simulink library "animation_cl"  (R2018b)
settings: Solver=VariableStepAuto  StartTime=0.0  StopTime=10.0  RelTol=1e-3
values from neighbouring files (symbols this model uses):
  zenith = 90-elevation    [animation_init.m]
libraries: vrlib x3, eulAng2RotMat_ul x1, dspvision x1
settings Model: Creator=mcobb  LastModifiedBy=mcobb

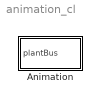
== system animation_cl ==
  Animation : Subsystem  mask{animSampleTime=0.1, elevation=75, radius=400, vidLogEnbl=on, vidDims=[240 480]}
      mask prompts: animSampleTime "Animation Sample Time"; vidLogEnbl "Enable"; vidDims "Video Dimensions"
      mask init:
      | animation_init
      mask DialogControl ParameterGroupVar Prompt: Viewpoint Specification
      mask DialogControl Container3 Prompt: Video File Logging

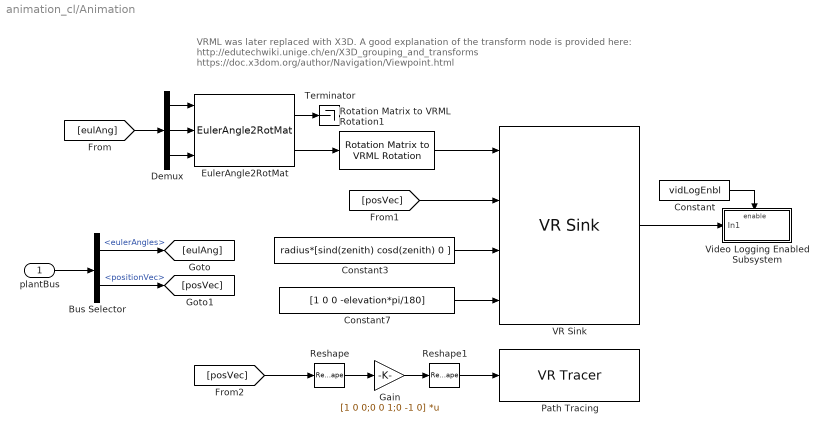
== system animation_cl/Animation ==
  note: VRML was later replaced with X3D. A good explanation of the transform node is provided here:
      | http://edutechwiki.unige.ch/en/X3D_grouping_and_transforms
      | https://doc.x3dom.org/author/Navigation/Viewpoint.html
  plantBus : Inport  OutDataTypeStr=Bus: plantBus
  Bus Selector : BusSelector  OutputSignals=eulerAngles,positionVec
  Constant : Constant  Value=vidLogEnbl
  Constant3 : Constant  Value=radius*[sind(zenith) cosd(zenith) 0 ]
  Constant7 : Constant  Value=[1 0 0 -elevation*pi/180]
  Demux : Demux  Outputs=3
  EulerAngle2RotMat : eulAng2RotMat_ul/EulerAngle2RotMat  SystemSampleTime=-1
  Gain : Gain  Gain=[1 0 0;0 0 1;0 -1 0]  Multiplication=Matrix(K*u)
  Path Tracing : vrlib/VR Tracer  VrmlFile=worldFile.wrl  MarkerName=Sphere  UseLines=on  UseTriads=off  MarkerScale=[1 1 1]*0.1  MarkerColorSelection=Selected from color list  MarkerColor=red  rgbval=[1 0 0]  Ts=1  ForceViewerOpen=off  ConnectPlane=off  PlaneCoeff=[0 1 0 0]  ConnectPoint=None  PointCoord=[0 0 0]
      settings: SourceProductName=Simulink 3D Animation  SourceProductBaseCode=VR
  Reshape : Reshape  OutputDimensionality=Column vector (2-D)
  Reshape1 : Reshape
  Rotation Matrix to VRML Rotation1 : vrlib/Utilities/Rotation Matrix to VRML Rotation  maxzero=1e-12
      settings: SourceProductName=Simulink 3D Animation  SourceProductBaseCode=VR
  Terminator : Terminator
  VR Sink : vrlib/VR Sink  InstantiateOnLoad=on  SampleTime=0.1  ViewEnable=on  RemoteChange=off  RemoteView=off  FieldsWritten=GND2BDY.rotation.4.1.1.double#GND2BDY.translation.3.1.1.double#VRML2CAM.translation.3.1.1.double#TRNS1.rotation.4.1.1.double  WorldFileName=worldFile.wrl  AutoView=on  VideoDimensions=[240 480]  AllowVariableSize=off  FigureProperties="{'Position', 'Name', 'Viewpoint', 'CameraBound', 'CameraDirection', 'CameraPosition', 'CameraUpVector', 'ZoomFactor', 'Antialiasing', 'Headlight', 'Lighting', 'NavPanel', 'Sound', 'StatusBar', 'Stereo3D', 'Stereo3DCameraOffset', 'Stereo3DHIT', 'ToolBar', 'Textures', 'Transparency', 'Triad', 'Wireframe', 'NavZones', 'NavMode', 'NavSpeed', 'CaptureFileFormat', 'CaptureFileName', 'Record2DCompressMethod', 'Record2DCompressQuality', 'Record2D', 'Record2DFileName', 'Record2DFPS'; [9.6200000000000000e+02   8.4000000000000000e+01   9.5800000000000000e+02   9.0400000000000000e+02], 'AWE or MHK System', 'Tracking', 'on', [9.4108294567115752e-02   0.0000000000000000e+00  -9.9556196637560901e-01], [-2.6473165272443846e+00   0.0000000000000000e+00   6.5099314699384685e+00], [0.0000000000000000e+00   1.0000000000000000e+00   0.0000000000000000e+00], [1.0000000000000000e+00], 'on', 'on', 'on', 'halfbar', 'on', 'on', 'off', [1.0000000149011612e-01], [0.0000000000000000e+00], 'on', 'on', 'on', 'none', 'off', 'off', 'fly', 'normal', 'tif', '%f_anim_%n.tif', 'auto', [7.5000000000000000e+01], 'off', '%f_anim_%n.avi', 'auto'}"
      settings: SourceProductBaseCode=VR
  Video Logging Enabled Subsystem : Subsystem
  wires:
  [eulAng] -> Demux/1
  Bus Selector/2 -> [posVec]  "<positionVec>"
  Bus Selector/1 -> [eulAng]  "<eulerAngles>"
  plantBus/1 -> Bus Selector/1
  EulerAngle2RotMat/1 -> Terminator/1
  Demux/2 -> EulerAngle2RotMat/2
  EulerAngle2RotMat/2 -> Rotation Matrix to VRML Rotation1/1
  Demux/3 -> EulerAngle2RotMat/3
  Demux/1 -> EulerAngle2RotMat/1
  Rotation Matrix to VRML Rotation1/1 -> VR Sink/1
  [posVec] -> VR Sink/2
  Constant3/1 -> VR Sink/3
  Constant7/1 -> VR Sink/4
  VR Sink/1 -> Video Logging Enabled Subsystem/1(In1)
  Constant/1 -> Video Logging Enabled Subsystem/Enable
  [posVec] -> Reshape/1
  Reshape/1 -> Gain/1
  Gain/1 -> Reshape1/1
  Reshape1/1 -> Path Tracing/1

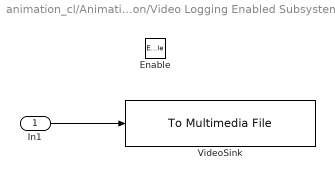
== system animation_cl/Animation/Video Logging Enabled Subsystem ==
  In1 : Inport
  Enable : EnablePort
  VideoSink : dspvision/To Multimedia File  outputFilename=outputVideo.avi  streamSelection=Video only  videoCompressor=MJPEG Compressor  audioCompressor=None (uncompressed)  imagePorts=One multidimensional signal  fileType=AVI  audioDatatype=Determine from input data type  fourcc=RGB  videoQuality=75  mj2000CompFactor=10
      settings: SourceProductName=Computer Vision System Toolbox  SourceProductBaseCode=VP
  wires:
  In1/1 -> VideoSink/1
